simulink model "StrapDownSim_Modified"  (R2013a)
settings: Solver=ode45  StartTime=0.0  StopTime=10  RelTol=1e-3
libraries: simulink_extras x6, aerolibnav x2
settings Model: Creator=Administrator  LastModifiedBy=Ibrahim_B92

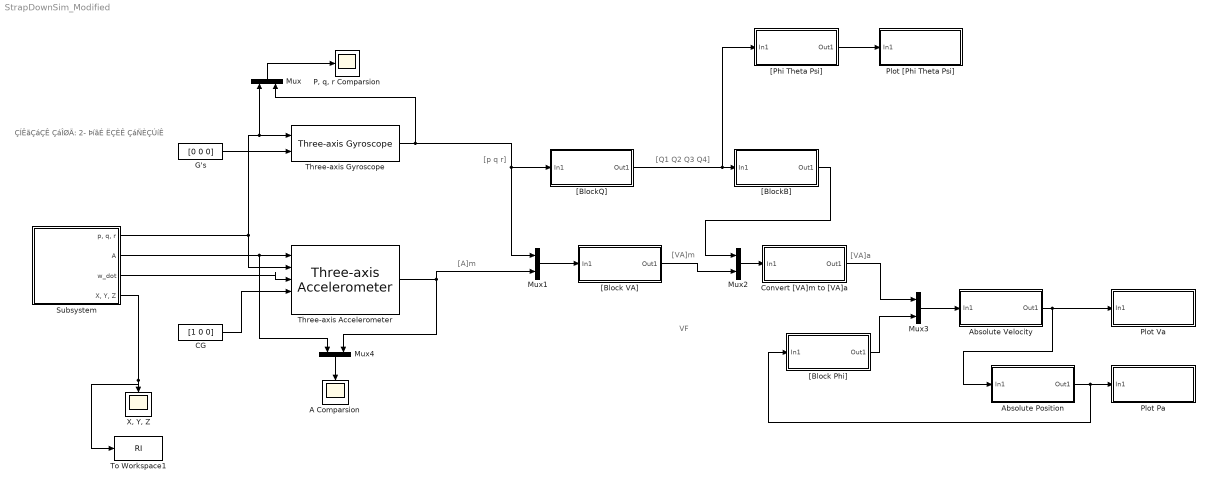
== system StrapDownSim_Modified ==
  note: [VA]a
  note: [VA]m
  note: VF
  note: [A]m
  note: [Q1 Q2 Q3 Q4]
  note: [p q r]
  note: ÇÍÊãÇáÇÊ ÇáÎØÃ:
      | 2- ÞíãÉ ËÇÈÊ ÇáÑÈÇÚíÊ
  A Comparsion : Scope
      settings: TimeRange=3  YMin=-30  YMax=10
  Absolute Position : Subsystem
  Absolute Velocity : Subsystem
  CG : Constant  Value=[1 0 0]
  Convert [VA]m to [VA]a : Subsystem  TreatAsAtomicUnit=on
  G's : Constant  Value=[0 0 0]
  Mux{,1..4} (5 alike) : Mux  Inputs=2
  "P, q, r Comparsion" : Scope
      settings: YMin=-0.6  YMax=0.8  SaveName=ScopeData2
  "Plot Pa " : Subsystem  TreatAsAtomicUnit=on
  Plot Va : Subsystem  TreatAsAtomicUnit=on
  Plot [Phi Theta Psi] : Subsystem  TreatAsAtomicUnit=on
  Subsystem : Subsystem
  Three-axis Accelerometer : aerolibnav/Three-axis Accelerometer  units=Metric (MKS)  acc=[1 0 0]  gtype=on  dtype_a=on  w_a=190  z_a=0.707  a_sf_cc=[1 0 0; 0 1 0; 0 0 1]  a_bias=[0 0 0]  a_rand=on  a_seeds=[23093 23094 23095]  a_pow=[0.0001 0.0001 0.0001]  a_sat="[-inf  -inf  -inf  inf inf inf]"  a_Ts=0
  Three-axis Gyroscope : aerolibnav/Three-axis Gyroscope  dtype_g=on  w_g=190  z_g=0.707  g_sf_cc=[1 0 0; 0 1 0; 0 0 1]  g_bias=[0 0 0]  g_sen=[0 0 0]  g_rand=on  g_seeds=[23093 23094 23095]  g_pow=[0.00005 0.00005 0.00005]  g_sat="[-inf  -inf  -inf  inf inf inf]"  g_Ts=0
  To Workspace1 : ToWorkspace  VariableName=RI  SampleTime=-1
      settings: Decimation=3
  "X, Y, Z" : Scope
      settings: TimeRange=3  YMin=-30  YMax=10  SaveName=ScopeData5
  "[Block Phi]" : Subsystem  TreatAsAtomicUnit=on
  "[Block VA]" : Subsystem  TreatAsAtomicUnit=on
  "[BlockB]" : Subsystem  TreatAsAtomicUnit=on
  "[BlockQ]" : Subsystem  TreatAsAtomicUnit=on
  "[Phi Theta Psi]" : Subsystem  TreatAsAtomicUnit=on
  wires:
  "[BlockB]"/1(Out1) -> Mux2/1
  "[BlockQ]"/1(Out1) -> "[Phi Theta Psi]"/1(In1), "[BlockB]"/1(In1)
  Mux1/1 -> "[Block VA]"/1(In1)
  "[Block VA]"/1(Out1) -> Mux2/2
  "[Block Phi]"/1(Out1) -> Mux3/2
  Mux2/1 -> Convert [VA]m to [VA]a/1(In1)
  Convert [VA]m to [VA]a/1(Out1) -> Mux3/1
  Mux3/1 -> Absolute Velocity/1(In1)
  Absolute Velocity/1(Out1) -> Plot Va/1(In1), Absolute Position/1(In1)
  "[Phi Theta Psi]"/1(Out1) -> Plot [Phi Theta Psi]/1(In1)
  Absolute Position/1(Out1) -> "[Block Phi]"/1(In1), "Plot Pa "/1(In1)
  Subsystem/1("p, q, r") -> Three-axis Gyroscope/1, Mux/1, Three-axis Accelerometer/2
  Subsystem/3(w_dot) -> Three-axis Accelerometer/3
  CG/1 -> Three-axis Accelerometer/4
  G's/1 -> Three-axis Gyroscope/2
  Three-axis Gyroscope/1 -> Mux1/1, "[BlockQ]"/1(In1), Mux/2
  Mux/1 -> "P, q, r Comparsion"/1
  Mux4/1 -> A Comparsion/1
  Subsystem/2(A) -> Mux4/1, Three-axis Accelerometer/1
  Three-axis Accelerometer/1 -> Mux1/2, Mux4/2
  Subsystem/4("X, Y, Z") -> To Workspace1/1, "X, Y, Z"/1

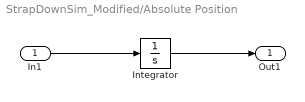
== system StrapDownSim_Modified/Absolute Position ==
  In1 : Inport
  Integrator : Integrator
  Out1 : Outport
  wires:
  In1/1 -> Integrator/1
  Integrator/1 -> Out1/1

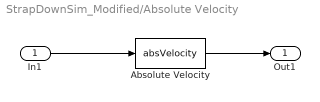
== system StrapDownSim_Modified/Absolute Velocity ==
  In1 : Inport
  Absolute Velocity : MATLABFcn  MATLABFcn=absVelocity  OutputDimensions=3
  Out1 : Outport
  wires:
  In1/1 -> Absolute Velocity/1
  Absolute Velocity/1 -> Out1/1

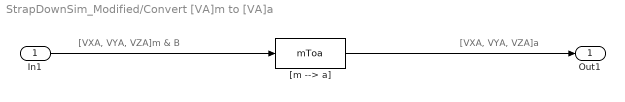
== system StrapDownSim_Modified/Convert [VA]m to [VA]a ==
  note: [VXA, VYA, VZA]m & B
  note: [VXA, VYA, VZA]a
  In1 : Inport
  "[m --> a]" : MATLABFcn  MATLABFcn=mToa  OutputDimensions=3
  Out1 : Outport
  wires:
  In1/1 -> "[m --> a]"/1
  "[m --> a]"/1 -> Out1/1

== system StrapDownSim_Modified/Plot Pa  ==
  In1 : Inport
  X : Scope
  wires:
  In1/1 -> X/1

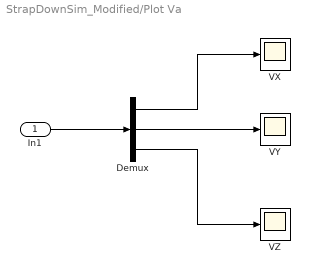
== system StrapDownSim_Modified/Plot Va ==
  In1 : Inport
  Demux : Demux  Outputs=3
  VX : Scope
  VY : Scope
      settings: SaveName=ScopeData3
  VZ : Scope
      settings: SaveName=ScopeData4
  wires:
  In1/1 -> Demux/1
  Demux/1 -> VX/1
  Demux/2 -> VY/1
  Demux/3 -> VZ/1

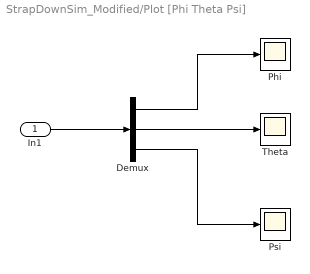
== system StrapDownSim_Modified/Plot [Phi Theta Psi] ==
  In1 : Inport
  Demux : Demux  Outputs=3
  Phi : Scope
  Psi : Scope
      settings: SaveName=ScopeData4
  Theta : Scope
      settings: SaveName=ScopeData3
  wires:
  In1/1 -> Demux/1
  Demux/1 -> Phi/1
  Demux/2 -> Theta/1
  Demux/3 -> Psi/1

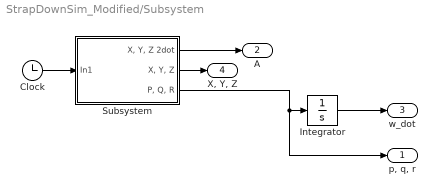
== system StrapDownSim_Modified/Subsystem ==
  Clock : Clock
  Integrator : Integrator
  Subsystem : Subsystem
  "p, q, r" : Outport
  A : Outport  Port=2
  w_dot : Outport  Port=3
  "X, Y, Z" : Outport  Port=4
  wires:
  Clock/1 -> Subsystem/1(In1)
  Subsystem/3("P, Q, R") -> Integrator/1, "p, q, r"/1
  Integrator/1 -> w_dot/1
  Subsystem/1("X, Y, Z 2dot") -> A/1
  Subsystem/2("X, Y, Z") -> "X, Y, Z"/1

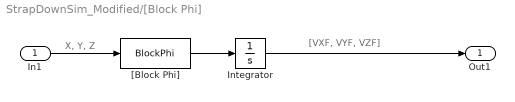
== system StrapDownSim_Modified/[Block Phi] ==
  note: X, Y, Z
  note: [VXF, VYF, VZF]
  In1 : Inport
  Integrator : Integrator
  "[Block Phi]" : MATLABFcn  MATLABFcn=BlockPhi  OutputDimensions=3
  Out1 : Outport
  wires:
  "[Block Phi]"/1 -> Integrator/1
  Integrator/1 -> Out1/1
  In1/1 -> "[Block Phi]"/1

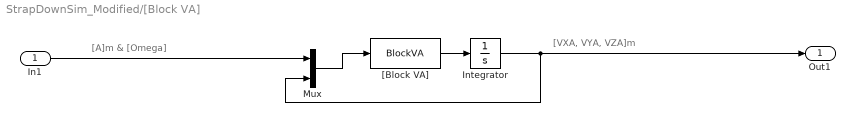
== system StrapDownSim_Modified/[Block VA] ==
  note: [A]m & [Omega]
  note: [VXA, VYA, VZA]m
  In1 : Inport
  Integrator : Integrator
  Mux : Mux  Inputs=2
  "[Block VA]" : MATLABFcn  MATLABFcn=BlockVA  OutputDimensions=3
  Out1 : Outport
  wires:
  In1/1 -> Mux/1
  "[Block VA]"/1 -> Integrator/1
  Mux/1 -> "[Block VA]"/1
  Integrator/1 -> Out1/1, Mux/2

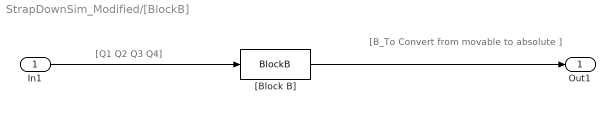
== system StrapDownSim_Modified/[BlockB] ==
  note: [Q1 Q2 Q3 Q4]
  note: [B_To Convert from movable to absolute ]
  In1 : Inport
  "[Block B]" : MATLABFcn  MATLABFcn=BlockB  OutputDimensions=9
  Out1 : Outport
  wires:
  In1/1 -> "[Block B]"/1
  "[Block B]"/1 -> Out1/1

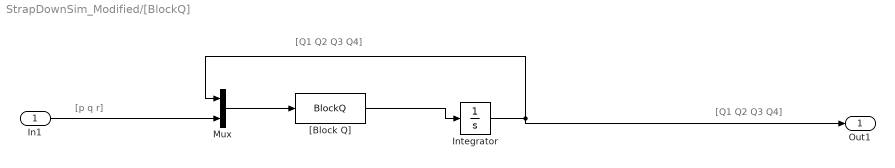
== system StrapDownSim_Modified/[BlockQ] ==
  note: [p q r]
  note: [Q1 Q2 Q3 Q4]
  note: [Q1 Q2 Q3 Q4]
  In1 : Inport
  Integrator : Integrator  InitialCondition=[0 0 0 1]
  Mux : Mux  Inputs=2
  "[Block Q]" : MATLABFcn  MATLABFcn=BlockQ  OutputDimensions=4
  Out1 : Outport
  wires:
  "[Block Q]"/1 -> Integrator/1
  Integrator/1 -> Mux/1, Out1/1
  Mux/1 -> "[Block Q]"/1
  In1/1 -> Mux/2

== system StrapDownSim_Modified/[Phi Theta Psi] ==
  note: [B]
  note: [Phi Theta Psi ]
  In1 : Inport
  "[phiTpsi]" : MATLABFcn  MATLABFcn=phiTpsi  OutputDimensions=3
  Out1 : Outport
  wires:
  In1/1 -> "[phiTpsi]"/1
  "[phiTpsi]"/1 -> Out1/1

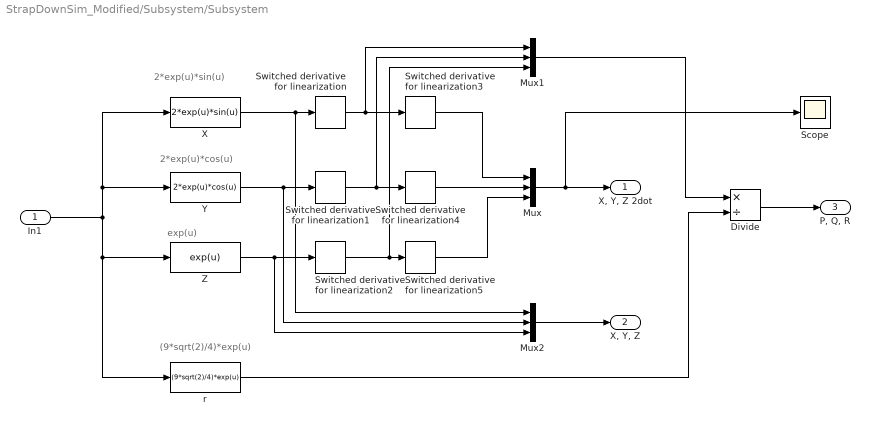
== system StrapDownSim_Modified/Subsystem/Subsystem ==
  note: (9*sqrt(2)/4)*exp(u)
  note: exp(u)
  note: 2*exp(u)*cos(u)
  note: 2*exp(u)*sin(u)
  In1 : Inport
  Divide : Product  Inputs=*/
  Mux : Mux  Inputs=3
  Mux1 : Mux  Inputs=3
  Mux2 : Mux  Inputs=3
  Scope : Scope
      settings: YMin=-50000  YMax=800000  SaveName=ScopeData6
  Switched derivative for linearization{,1..5} (6 alike) : simulink_extras/Linearization/Switched derivative for linearization  switchVal=1  derivConst=1
  X : MATLABFcn  MATLABFcn=2*exp(u)*sin(u)
  Y : MATLABFcn  MATLABFcn=2*exp(u)*cos(u)
  Z : MATLABFcn  MATLABFcn=exp(u)
  r : MATLABFcn  MATLABFcn=(9*sqrt(2)/4)*exp(u)
  "X, Y, Z 2dot" : Outport
  "X, Y, Z" : Outport  Port=2
  "P, Q, R" : Outport  Port=3
  wires:
  In1/1 -> X/1, Y/1, Z/1, r/1
  X/1 -> Switched derivative for linearization/1, Mux2/1
  Y/1 -> Switched derivative for linearization1/1, Mux2/2
  Z/1 -> Switched derivative for linearization2/1, Mux2/3
  Switched derivative for linearization/1 -> Switched derivative for linearization3/1, Mux1/1
  Switched derivative for linearization1/1 -> Switched derivative for linearization4/1, Mux1/2
  Switched derivative for linearization2/1 -> Switched derivative for linearization5/1, Mux1/3
  Mux1/1 -> Divide/1
  Mux/1 -> Scope/1, "X, Y, Z 2dot"/1
  Switched derivative for linearization3/1 -> Mux/1
  Switched derivative for linearization4/1 -> Mux/2
  Switched derivative for linearization5/1 -> Mux/3
  Mux2/1 -> "X, Y, Z"/1
  r/1 -> Divide/2
  Divide/1 -> "P, Q, R"/1
